simulink model "building_EXAMPLE_v1"  (R2016b)
settings: Solver=ode23tb  StartTime=-building.preruntime+8760*3600  StopTime=building.runtime+8760*3600  MaxStep=600  EnableMultiTasking=on
StartFcn:
  | tic
StopFcn:
  | toc
values from neighbouring files (symbols this model uses):
  building = create_building_automatic(building, modify, import_mode, name_XML, name_EXCEL, name_PHPP, NUMBEROFZONES)    [work_EXAMPLE_v1.m]
undefined symbols (not defined in the file or in its folder): A, B, C, cp, Dd, Dreifach, FluidMix, get_building, ID, MassFlow, p, Pressure, Qdot_C, Qdot_C_energy, Qdot_H, Qdot_H_energy, Qdot_I_electricity, Qdot_I_electricity_energy, Qdot_I_light, Qdot_I_light_energy, Qdot_I_person, Qdot_I_person_energy, Qdot_S, Qdot_S_energy, Qdot_T_ground, Qdot_T_ground_energy, Qdot_T_neighbour, Qdot_T_neighbour_energy, Qdot_T_opaque, Qdot_T_opaque_energy, Qdot_T_window, Qdot_T_window_energy, Qdot_V_infiltration, Qdot_V_infiltration_energy, Qdot_V_mech, Qdot_V_mech_energy, Qdot_V_window, Qdot_V_window_energy, rho, Tc, Temperature, Tr, Ts, Wärmeschutzglas, x_CO2, x_H2O, x_VOC
libraries: carnotUIBK x1931, carnot x83, simulink_extras x22, simulink x12
(part 2 of 35)

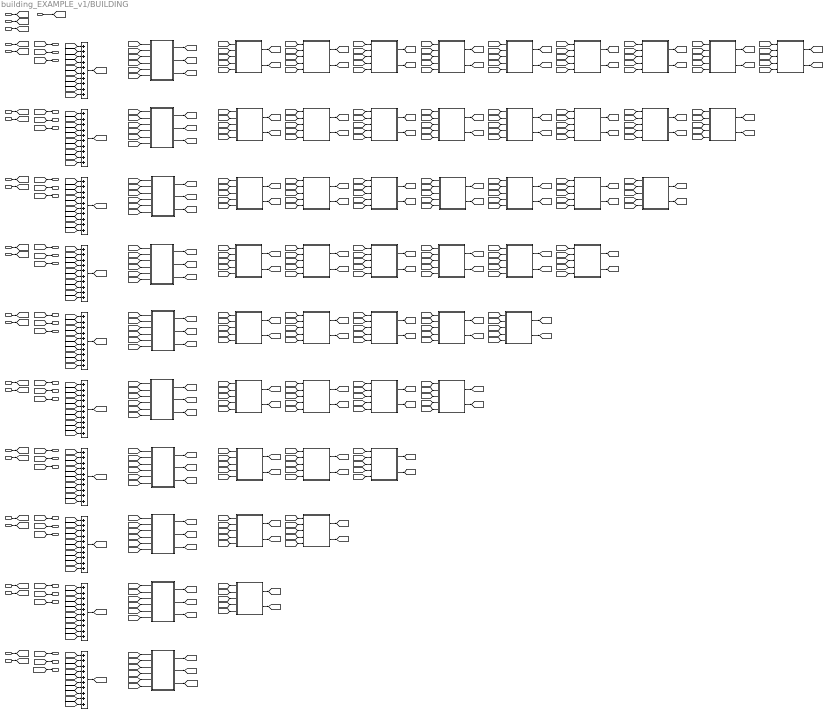
== system building_EXAMPLE_v1/BUILDING ==
  note: INTERSECTION 1_2
  note: ZONE 1 - SUM UP S
  note: ZONE 6 - INPUT AND OUTPUT
  note: ZONE 5 - INPUT AND OUTPUT
  note: ZONE 4 - INPUT AND OUTPUT
  note: ZONE 3 - INPUT AND OUTPUT
  note: ZONE 2 - INPUT AND OUTPUT
  note: ZONE 1 - INPUT AND OUTPUT
  note: BUS BOUNDARY
  note: ZONE 2 - SUM UP S
  note: ZONE 3 - SUM UP S
  note: ZONE 4 - SUM UP S
  note: ZONE 5 - SUM UP S
  note: ZONE 6 - SUM UP S
  note: ZONE 7 - INPUT AND OUTPUT
  note: ZONE 7 - SUM UP S
  note: ZONE 8 - INPUT AND OUTPUT
  note: ZONE 8 - SUM UP S
  note: ZONE 9 - INPUT AND OUTPUT
  note: ZONE 9 - SUM UP S
  note: ZONE 10 - INPUT AND OUTPUT
  note: ZONE 10 - SUM UP S
  note: ZONE 2
  note: ZONE 3
  note: ZONE 4
  note: ZONE 5
  note: ZONE6
  note: ZONE 7
  note: ZONE 8
  note: ZONE 9
  note: ZONE 10
  note: CONTROL
  note: INTERSECTION 1_10
  note: INTERSECTION 1_3
  note: INTERSECTION 1_4
  note: INTERSECTION 1_5
  note: INTERSECTION 1_6
  note: INTERSECTION 1_7
  note: INTERSECTION 1_8
  note: INTERSECTION 1_9
  note: INTERSECTION 2_3
  note: INTERSECTION 2_9
  note: INTERSECTION 2_10
  note: INTERSECTION 2_4
  note: INTERSECTION 2_5
  note: INTERSECTION 2_6
  note: INTERSECTION 2_7
  note: INTERSECTION 2_8
  note: INTERSECTION 3_4
  note: INTERSECTION 3_5
  note: INTERSECTION 3_6
  note: INTERSECTION 3_7
  note: INTERSECTION 3_8
  note: INTERSECTION 3_9
  note: INTERSECTION 3_10
  note: INTERSECTION 4_5
  note: INTERSECTION 4_6
  note: INTERSECTION 4_7
  note: INTERSECTION 4_8
  note: INTERSECTION 4_9
  note: INTERSECTION 4_10
  note: INTERSECTION 5_6
  note: INTERSECTION 5_7
  note: INTERSECTION 5_8
  note: INTERSECTION 5_9
  note: INTERSECTION 5_10
  note: INTERSECTION 6_7
  note: INTERSECTION 6_8
  note: INTERSECTION 6_9
  note: INTERSECTION 6_10
  note: INTERSECTION 7_8
  note: INTERSECTION 7_9
  note: INTERSECTION 7_10
  note: INTERSECTION 8_9
  note: INTERSECTION 8_10
  note: INTERSECTION 9_10
  note: ZONE 1
  WDB : Inport
  GDB : Inport  Port=2
  NDB : Inport  Port=3
  S_HVAC[1] : Inport  Port=4
  qdot_in[1] : Inport  Port=5
  S_HVAC[2] : Inport  Port=6
  qdot_in[2] : Inport  Port=7
  S_HVAC[3] : Inport  Port=8
  qdot_in[3] : Inport  Port=9
  S_HVAC[4] : Inport  Port=10
  qdot_in[4] : Inport  Port=11
  S_HVAC[5] : Inport  Port=12
  qdot_in[5] : Inport  Port=13
  S_HVAC[6] : Inport  Port=14
  qdot_in[6] : Inport  Port=15
  S_HVAC[7] : Inport  Port=16
  qdot_in[7] : Inport  Port=17
  S_HVAC[8] : Inport  Port=18
  qdot_in[8] : Inport  Port=19
  S_HVAC[9] : Inport  Port=20
  qdot_in[9] : Inport  Port=21
  S_HVAC[10] : Inport  Port=22
  qdot_in[10] : Inport  Port=23
  control : Inport  Port=24
  Add{,1..9} (10 alike) : Sum  Inputs=++++++++++
  INTERSECTION_1_10 : Subsystem  VariantControl=Variant1  mask{intersection=b.thermalzone.intersection{1,10}}
      mask prompts: intersection "INTERSECTION object"
      mask init:
      | i = intersection;
      | z = intersection;
      mask Display: fprintf('%s',intersection.name)
  INTERSECTION_1_2 : Subsystem  VariantControl=Variant1  mask{intersection=b.thermalzone.intersection{1,2}}
      mask prompts: intersection "INTERSECTION object"
      mask init:
      | i = intersection;
      | z = intersection;
      mask Display: fprintf('%s',intersection.name)
  INTERSECTION_1_3 : Subsystem  VariantControl=Variant1  mask{intersection=b.thermalzone.intersection{1,3}}
      mask prompts: intersection "INTERSECTION object"
      mask init:
      | i = intersection;
      | z = intersection;
      mask Display: fprintf('%s',intersection.name)
  INTERSECTION_1_4 : Subsystem  VariantControl=Variant1  mask{intersection=b.thermalzone.intersection{1,4}}
      mask prompts: intersection "INTERSECTION object"
      mask init:
      | i = intersection;
      | z = intersection;
      mask Display: fprintf('%s',intersection.name)
  INTERSECTION_1_5 : Subsystem  VariantControl=Variant1  mask{intersection=b.thermalzone.intersection{1,5}}
      mask prompts: intersection "INTERSECTION object"
      mask init:
      | i = intersection;
      | z = intersection;
      mask Display: fprintf('%s',intersection.name)
  INTERSECTION_1_6 : Subsystem  VariantControl=Variant1  mask{intersection=b.thermalzone.intersection{1,6}}
      mask prompts: intersection "INTERSECTION object"
      mask init:
      | i = intersection;
      | z = intersection;
      mask Display: fprintf('%s',intersection.name)
  INTERSECTION_1_7 : Subsystem  VariantControl=Variant1  mask{intersection=b.thermalzone.intersection{1,7}}
      mask prompts: intersection "INTERSECTION object"
      mask init:
      | i = intersection;
      | z = intersection;
      mask Display: fprintf('%s',intersection.name)
  INTERSECTION_1_8 : Subsystem  VariantControl=Variant1  mask{intersection=b.thermalzone.intersection{1,8}}
      mask prompts: intersection "INTERSECTION object"
      mask init:
      | i = intersection;
      | z = intersection;
      mask Display: fprintf('%s',intersection.name)
  INTERSECTION_1_9 : Subsystem  VariantControl=Variant1  mask{intersection=b.thermalzone.intersection{1,9}}
      mask prompts: intersection "INTERSECTION object"
      mask init:
      | i = intersection;
      | z = intersection;
      mask Display: fprintf('%s',intersection.name)
  INTERSECTION_2_10 : Subsystem  VariantControl=Variant1  mask{intersection=b.thermalzone.intersection{2,10}}
      mask prompts: intersection "INTERSECTION object"
      mask init:
      | i = intersection;
      | z = intersection;
      mask Display: fprintf('%s',intersection.name)
  INTERSECTION_2_3 : Subsystem  VariantControl=Variant1  mask{intersection=b.thermalzone.intersection{2,3}}
      mask prompts: intersection "INTERSECTION object"
      mask init:
      | i = intersection;
      | z = intersection;
      mask Display: fprintf('%s',intersection.name)
  INTERSECTION_2_4 : Subsystem  VariantControl=Variant1  mask{intersection=b.thermalzone.intersection{2,4}}
      mask prompts: intersection "INTERSECTION object"
      mask init:
      | i = intersection;
      | z = intersection;
      mask Display: fprintf('%s',intersection.name)
  INTERSECTION_2_5 : Subsystem  VariantControl=Variant1  mask{intersection=b.thermalzone.intersection{2,5}}
      mask prompts: intersection "INTERSECTION object"
      mask init:
      | i = intersection;
      | z = intersection;
      mask Display: fprintf('%s',intersection.name)
  INTERSECTION_2_6 : Subsystem  VariantControl=Variant1  mask{intersection=b.thermalzone.intersection{2,6}}
      mask prompts: intersection "INTERSECTION object"
      mask init:
      | i = intersection;
      | z = intersection;
      mask Display: fprintf('%s',intersection.name)
  INTERSECTION_2_7 : Subsystem  VariantControl=Variant1  mask{intersection=b.thermalzone.intersection{2,7}}
      mask prompts: intersection "INTERSECTION object"
      mask init:
      | i = intersection;
      | z = intersection;
      mask Display: fprintf('%s',intersection.name)
  INTERSECTION_2_8 : Subsystem  VariantControl=Variant1  mask{intersection=b.thermalzone.intersection{2,8}}
      mask prompts: intersection "INTERSECTION object"
      mask init:
      | i = intersection;
      | z = intersection;
      mask Display: fprintf('%s',intersection.name)
  INTERSECTION_2_9 : Subsystem  VariantControl=Variant1  mask{intersection=b.thermalzone.intersection{2,9}}
      mask prompts: intersection "INTERSECTION object"
      mask init:
      | i = intersection;
      | z = intersection;
      mask Display: fprintf('%s',intersection.name)
  INTERSECTION_3_10 : Subsystem  VariantControl=Variant1  mask{intersection=b.thermalzone.intersection{3,10}}
      mask prompts: intersection "INTERSECTION object"
      mask init:
      | i = intersection;
      | z = intersection;
      mask Display: fprintf('%s',intersection.name)
  INTERSECTION_3_4 : Subsystem  VariantControl=Variant1  mask{intersection=b.thermalzone.intersection{3,4}}
      mask prompts: intersection "INTERSECTION object"
      mask init:
      | i = intersection;
      | z = intersection;
      mask Display: fprintf('%s',intersection.name)
  INTERSECTION_3_5 : Subsystem  VariantControl=Variant1  mask{intersection=b.thermalzone.intersection{3,5}}
      mask prompts: intersection "INTERSECTION object"
      mask init:
      | i = intersection;
      | z = intersection;
      mask Display: fprintf('%s',intersection.name)
  INTERSECTION_3_6 : Subsystem  VariantControl=Variant1  mask{intersection=b.thermalzone.intersection{3,6}}
      mask prompts: intersection "INTERSECTION object"
      mask init:
      | i = intersection;
      | z = intersection;
      mask Display: fprintf('%s',intersection.name)
  INTERSECTION_3_7 : Subsystem  VariantControl=Variant1  mask{intersection=b.thermalzone.intersection{3,7}}
      mask prompts: intersection "INTERSECTION object"
      mask init:
      | i = intersection;
      | z = intersection;
      mask Display: fprintf('%s',intersection.name)
  INTERSECTION_3_8 : Subsystem  VariantControl=Variant1  mask{intersection=b.thermalzone.intersection{3,8}}
      mask prompts: intersection "INTERSECTION object"
      mask init:
      | i = intersection;
      | z = intersection;
      mask Display: fprintf('%s',intersection.name)
  INTERSECTION_3_9 : Subsystem  VariantControl=Variant1  mask{intersection=b.thermalzone.intersection{3,9}}
      mask prompts: intersection "INTERSECTION object"
      mask init:
      | i = intersection;
      | z = intersection;
      mask Display: fprintf('%s',intersection.name)
  INTERSECTION_4_10 : Subsystem  VariantControl=Variant1  mask{intersection=b.thermalzone.intersection{4,10}}
      mask prompts: intersection "INTERSECTION object"
      mask init:
      | i = intersection;
      | z = intersection;
      mask Display: fprintf('%s',intersection.name)
  INTERSECTION_4_5 : Subsystem  VariantControl=Variant1  mask{intersection=b.thermalzone.intersection{4,5}}
      mask prompts: intersection "INTERSECTION object"
      mask init:
      | i = intersection;
      | z = intersection;
      mask Display: fprintf('%s',intersection.name)
  INTERSECTION_4_6 : Subsystem  VariantControl=Variant1  mask{intersection=b.thermalzone.intersection{4,6}}
      mask prompts: intersection "INTERSECTION object"
      mask init:
      | i = intersection;
      | z = intersection;
      mask Display: fprintf('%s',intersection.name)
  INTERSECTION_4_7 : Subsystem  VariantControl=Variant1  mask{intersection=b.thermalzone.intersection{4,7}}
      mask prompts: intersection "INTERSECTION object"
      mask init:
      | i = intersection;
      | z = intersection;
      mask Display: fprintf('%s',intersection.name)
  INTERSECTION_4_8 : Subsystem  VariantControl=Variant1  mask{intersection=b.thermalzone.intersection{4,8}}
      mask prompts: intersection "INTERSECTION object"
      mask init:
      | i = intersection;
      | z = intersection;
      mask Display: fprintf('%s',intersection.name)
  INTERSECTION_4_9 : Subsystem  VariantControl=Variant1  mask{intersection=b.thermalzone.intersection{4,9}}
      mask prompts: intersection "INTERSECTION object"
      mask init:
      | i = intersection;
      | z = intersection;
      mask Display: fprintf('%s',intersection.name)
  INTERSECTION_5_10 : Subsystem  VariantControl=Variant1  mask{intersection=b.thermalzone.intersection{5,10}}
      mask prompts: intersection "INTERSECTION object"
      mask init:
      | i = intersection;
      | z = intersection;
      mask Display: fprintf('%s',intersection.name)
  INTERSECTION_5_6 : Subsystem  VariantControl=Variant1  mask{intersection=b.thermalzone.intersection{5,6}}
      mask prompts: intersection "INTERSECTION object"
      mask init:
      | i = intersection;
      | z = intersection;
      mask Display: fprintf('%s',intersection.name)
  INTERSECTION_5_7 : Subsystem  VariantControl=Variant1  mask{intersection=b.thermalzone.intersection{5,7}}
      mask prompts: intersection "INTERSECTION object"
      mask init:
      | i = intersection;
      | z = intersection;
      mask Display: fprintf('%s',intersection.name)
  INTERSECTION_5_8 : Subsystem  VariantControl=Variant1  mask{intersection=b.thermalzone.intersection{5,8}}
      mask prompts: intersection "INTERSECTION object"
      mask init:
      | i = intersection;
      | z = intersection;
      mask Display: fprintf('%s',intersection.name)
  INTERSECTION_5_9 : Subsystem  VariantControl=Variant1  mask{intersection=b.thermalzone.intersection{5,9}}
      mask prompts: intersection "INTERSECTION object"
      mask init:
      | i = intersection;
      | z = intersection;
      mask Display: fprintf('%s',intersection.name)
  INTERSECTION_6_10 : Subsystem  VariantControl=Variant1  mask{intersection=b.thermalzone.intersection{6,10}}
      mask prompts: intersection "INTERSECTION object"
      mask init:
      | i = intersection;
      | z = intersection;
      mask Display: fprintf('%s',intersection.name)
  INTERSECTION_6_7 : Subsystem  VariantControl=Variant1  mask{intersection=b.thermalzone.intersection{6,7}}
      mask prompts: intersection "INTERSECTION object"
      mask init:
      | i = intersection;
      | z = intersection;
      mask Display: fprintf('%s',intersection.name)
  INTERSECTION_6_8 : Subsystem  VariantControl=Variant1  mask{intersection=b.thermalzone.intersection{6,8}}
      mask prompts: intersection "INTERSECTION object"
      mask init:
      | i = intersection;
      | z = intersection;
      mask Display: fprintf('%s',intersection.name)
  INTERSECTION_6_9 : Subsystem  VariantControl=Variant1  mask{intersection=b.thermalzone.intersection{6,9}}
      mask prompts: intersection "INTERSECTION object"
      mask init:
      | i = intersection;
      | z = intersection;
      mask Display: fprintf('%s',intersection.name)
  INTERSECTION_7_10 : Subsystem  VariantControl=Variant1  mask{intersection=b.thermalzone.intersection{7,10}}
      mask prompts: intersection "INTERSECTION object"
      mask init:
      | i = intersection;
      | z = intersection;
      mask Display: fprintf('%s',intersection.name)
  INTERSECTION_7_8 : Subsystem  VariantControl=Variant1  mask{intersection=b.thermalzone.intersection{7,8}}
      mask prompts: intersection "INTERSECTION object"
      mask init:
      | i = intersection;
      | z = intersection;
      mask Display: fprintf('%s',intersection.name)
  INTERSECTION_7_9 : Subsystem  VariantControl=Variant1  mask{intersection=b.thermalzone.intersection{7,9}}
      mask prompts: intersection "INTERSECTION object"
      mask init:
      | i = intersection;
      | z = intersection;
      mask Display: fprintf('%s',intersection.name)
  INTERSECTION_8_10 : Subsystem  VariantControl=Variant1  mask{intersection=b.thermalzone.intersection{8,10}}
      mask prompts: intersection "INTERSECTION object"
      mask init:
      | i = intersection;
      | z = intersection;
      mask Display: fprintf('%s',intersection.name)
  INTERSECTION_8_9 : Subsystem  VariantControl=Variant1  mask{intersection=b.thermalzone.intersection{8,9}}
      mask prompts: intersection "INTERSECTION object"
      mask init:
      | i = intersection;
      | z = intersection;
      mask Display: fprintf('%s',intersection.name)
  INTERSECTION_9_10 : Subsystem  VariantControl=Variant1  mask{intersection=b.thermalzone.intersection{9,10}}
      mask prompts: intersection "INTERSECTION object"
      mask init:
      | i = intersection;
      | z = intersection;
      mask Display: fprintf('%s',intersection.name)
  ZONE_1 : Subsystem  mask{zone=b.thermalzone.zone(1)}
      mask prompts: zone "ZONE object"
      mask init:
      | z = zone;
      mask Display: fprintf('%s',zone.name)
  ZONE_10 : Subsystem  mask{zone=b.thermalzone.zone(10)}
      mask prompts: zone "ZONE object"
      mask init:
      | z = zone;
      mask Display: fprintf('%s',zone.name)
  ZONE_2 : Subsystem  mask{zone=b.thermalzone.zone(2)}
      mask prompts: zone "ZONE object"
      mask init:
      | z = zone;
      mask Display: fprintf('%s',zone.name)
  ZONE_3 : Subsystem  mask{zone=b.thermalzone.zone(3)}
      mask prompts: zone "ZONE object"
      mask init:
      | z = zone;
      mask Display: fprintf('%s',zone.name)
  ZONE_4 : Subsystem  mask{zone=b.thermalzone.zone(4)}
      mask prompts: zone "ZONE object"
      mask init:
      | z = zone;
      mask Display: fprintf('%s',zone.name)
  ZONE_5 : Subsystem  mask{zone=b.thermalzone.zone(5)}
      mask prompts: zone "ZONE object"
      mask init:
      | z = zone;
      mask Display: fprintf('%s',zone.name)
  ZONE_6 : Subsystem  mask{zone=b.thermalzone.zone(6)}
      mask prompts: zone "ZONE object"
      mask init:
      | z = zone;
      mask Display: fprintf('%s',zone.name)
  ZONE_7 : Subsystem  mask{zone=b.thermalzone.zone(7)}
      mask prompts: zone "ZONE object"
      mask init:
      | z = zone;
      mask Display: fprintf('%s',zone.name)
  ZONE_8 : Subsystem  mask{zone=b.thermalzone.zone(8)}
      mask prompts: zone "ZONE object"
      mask init:
      | z = zone;
      mask Display: fprintf('%s',zone.name)
  ZONE_9 : Subsystem  mask{zone=b.thermalzone.zone(9)}
      mask prompts: zone "ZONE object"
      mask init:
      | z = zone;
      mask Display: fprintf('%s',zone.name)
  BDB[1] : Outport
  AIB[1] : Outport  Port=2
  theta_out[1] : Outport  Port=3
  BDB[2] : Outport  Port=4
  AIB[2] : Outport  Port=5
  theta_out[2] : Outport  Port=6
  BDB[3] : Outport  Port=7
  AIB[3] : Outport  Port=8
  theta_out[3] : Outport  Port=9
  BDB[4] : Outport  Port=10
  AIB[4] : Outport  Port=11
  theta_out[4] : Outport  Port=12
  BDB[5] : Outport  Port=13
  AIB[5] : Outport  Port=14
  theta_out[5] : Outport  Port=15
  BDB[6] : Outport  Port=16
  AIB[6] : Outport  Port=17
  theta_out[6] : Outport  Port=18
  BDB[7] : Outport  Port=19
  AIB[7] : Outport  Port=20
  theta_out[7] : Outport  Port=21
  BDB[8] : Outport  Port=22
  AIB[8] : Outport  Port=23
  theta_out[8] : Outport  Port=24
  BDB[9] : Outport  Port=25
  AIB[9] : Outport  Port=26
  theta_out[9] : Outport  Port=27
  BDB[10] : Outport  Port=28
  AIB[10] : Outport  Port=29
  theta_out[10] : Outport  Port=30
  wires:
  WDB/1 -> [WDB]
  GDB/1 -> [GDB]
  NDB/1 -> [NDB]
  S_HVAC[1]/1 -> [S_HVAC_1]
  qdot_in[1]/1 -> [qdot_in_1]
  [BDB_1] -> BDB[1]/1
  [AIB_1] -> AIB[1]/1
  [theta_out_1] -> theta_out[1]/1
  S_HVAC[2]/1 -> [S_HVAC_2]
  qdot_in[2]/1 -> [qdot_in_2]
  qdot_in[3]/1 -> [qdot_in_3]
  S_HVAC[3]/1 -> [S_HVAC_3]
  S_HVAC[4]/1 -> [S_HVAC_4]
  qdot_in[4]/1 -> [qdot_in_4]
  S_HVAC[5]/1 -> [S_HVAC_5]
  qdot_in[5]/1 -> [qdot_in_5]
  qdot_in[6]/1 -> [qdot_in_6]
  S_HVAC[6]/1 -> [S_HVAC_6]
  [BDB_2] -> BDB[2]/1
  [AIB_2] -> AIB[2]/1
  [theta_out_2] -> theta_out[2]/1
  [BDB_3] -> BDB[3]/1
  [AIB_3] -> AIB[3]/1
  [theta_out_3] -> theta_out[3]/1
  [BDB_4] -> BDB[4]/1
  [AIB_4] -> AIB[4]/1
  [theta_out_4] -> theta_out[4]/1
  [BDB_5] -> BDB[5]/1
  [AIB_5] -> AIB[5]/1
  [theta_out_5] -> theta_out[5]/1
  [BDB_6] -> BDB[6]/1
  [AIB_6] -> AIB[6]/1
  [theta_out_6] -> theta_out[6]/1
  [S_HVAC_1] -> Add/1
  [S_I_16] -> Add/6
  [S_I_12] -> Add/2
  [S_I_13] -> Add/3
  [S_I_14] -> Add/4
  [S_I_15] -> Add/5
  Add/1 -> [S_in_1]
  [S_HVAC_2] -> Add1/1
  Add1/1 -> [S_in_2]
  Add2/1 -> [S_in_3]
  Add3/1 -> [S_in_4]
  Add4/1 -> [S_in_5]
  Add5/1 -> [S_in_6]
  [S_I_17] -> Add/7
  [S_I_18] -> Add/8
  [S_I_19] -> Add/9
  [S_I_110] -> Add/10
  [S_I_27] -> Add1/7
  [S_I_28] -> Add1/8
  [S_I_29] -> Add1/9
  [S_I_210] -> Add1/10
  [S_I_21] -> Add1/2
  [S_I_23] -> Add1/3
  [S_I_26] -> Add1/6
  [S_I_25] -> Add1/5
  [S_I_24] -> Add1/4
  [S_I_37] -> Add2/7
  [S_I_38] -> Add2/8
  [S_I_39] -> Add2/9
  [S_I_310] -> Add2/10
  [S_HVAC_3] -> Add2/1
  [S_I_31] -> Add2/2
  [S_I_32] -> Add2/3
  [S_I_34] -> Add2/4
  [S_I_35] -> Add2/5
  [S_I_36] -> Add2/6
  [S_I_47] -> Add3/7
  [S_I_48] -> Add3/8
  [S_I_49] -> Add3/9
  [S_I_410] -> Add3/10
  [S_HVAC_4] -> Add3/1
  [S_I_41] -> Add3/2
  [S_I_42] -> Add3/3
  [S_I_43] -> Add3/4
  [S_I_45] -> Add3/5
  [S_I_46] -> Add3/6
  [S_I_57] -> Add4/7
  [S_I_58] -> Add4/8
  [S_I_59] -> Add4/9
  [S_I_510] -> Add4/10
  [S_HVAC_5] -> Add4/1
  [S_I_51] -> Add4/2
  [S_I_52] -> Add4/3
  [S_I_53] -> Add4/4
  [S_I_54] -> Add4/5
  [S_I_56] -> Add4/6
  [S_I_67] -> Add5/7
  [S_I_68] -> Add5/8
  [S_I_69] -> Add5/9
  [S_I_610] -> Add5/10
  [S_HVAC_6] -> Add5/1
  [S_I_61] -> Add5/2
  [S_I_62] -> Add5/3
  [S_I_63] -> Add5/4
  [S_I_64] -> Add5/5
  [S_I_65] -> Add5/6
  qdot_in[7]/1 -> [qdot_in_7]
  S_HVAC[7]/1 -> [S_HVAC_7]
  [BDB_7] -> BDB[7]/1
  [AIB_7] -> AIB[7]/1
  [theta_out_7] -> theta_out[7]/1
  Add6/1 -> [S_in_7]
  [S_I_76] -> Add6/7
  [S_I_78] -> Add6/8
  [S_I_79] -> Add6/9
  [S_I_710] -> Add6/10
  [S_HVAC_7] -> Add6/1
  [S_I_71] -> Add6/2
  [S_I_72] -> Add6/3
  [S_I_73] -> Add6/4
  [S_I_74] -> Add6/5
  [S_I_75] -> Add6/6
  qdot_in[8]/1 -> [qdot_in_8]
  S_HVAC[8]/1 -> [S_HVAC_8]
  [BDB_8] -> BDB[8]/1
  [AIB_8] -> AIB[8]/1
  [theta_out_8] -> theta_out[8]/1
  Add7/1 -> [S_in_8]
  [S_I_86] -> Add7/7
  [S_I_87] -> Add7/8
  [S_I_89] -> Add7/9
  [S_I_810] -> Add7/10
  [S_HVAC_8] -> Add7/1
  [S_I_81] -> Add7/2
  [S_I_82] -> Add7/3
  [S_I_83] -> Add7/4
  [S_I_84] -> Add7/5
  [S_I_85] -> Add7/6
  qdot_in[9]/1 -> [qdot_in_9]
  S_HVAC[9]/1 -> [S_HVAC_9]
  [BDB_9] -> BDB[9]/1
  [AIB_9] -> AIB[9]/1
  [theta_out_9] -> theta_out[9]/1
  Add8/1 -> [S_in_9]
  [S_I_96] -> Add8/7
  [S_I_97] -> Add8/8
  [S_I_98] -> Add8/9
  [S_I_910] -> Add8/10
  [S_HVAC_9] -> Add8/1
  [S_I_91] -> Add8/2
  [S_I_92] -> Add8/3
  [S_I_93] -> Add8/4
  [S_I_94] -> Add8/5
  [S_I_95] -> Add8/6
  qdot_in[10]/1 -> [qdot_in_10]
  S_HVAC[10]/1 -> [S_HVAC_10]
  [BDB_10] -> BDB[10]/1
  [AIB_10] -> AIB[10]/1
  [theta_out_10] -> theta_out[10]/1
  Add9/1 -> [S_in_10]
  [S_I_106] -> Add9/7
  [S_I_107] -> Add9/8
  [S_I_108] -> Add9/9
  [S_I_109] -> Add9/10
  [S_HVAC_10] -> Add9/1
  [S_I_101] -> Add9/2
  [S_I_102] -> Add9/3
  [S_I_103] -> Add9/4
  [S_I_104] -> Add9/5
  [S_I_105] -> Add9/6
  ZONE_2/1(BDB) -> [BDB_2]
  ZONE_2/2(AIB) -> [AIB_2]
  ZONE_2/3(theta_out) -> [theta_out_2z]
  [qdot_in_2] -> ZONE_2/5(Qdot_in)
  [S_in_2] -> ZONE_2/4(S_in)
  [GDB] -> ZONE_2/2(GDB)
  [WDB] -> ZONE_2/1(WDB)
  [NDB] -> ZONE_2/3(NDB)
  ZONE_3/1(BDB) -> [BDB_3]
  ZONE_3/2(AIB) -> [AIB_3]
  ZONE_3/3(theta_out) -> [theta_out_3z]
  [qdot_in_3] -> ZONE_3/5(Qdot_in)
  [S_in_3] -> ZONE_3/4(S_in)
  [GDB] -> ZONE_3/2(GDB)
  [WDB] -> ZONE_3/1(WDB)
  [NDB] -> ZONE_3/3(NDB)
  ZONE_4/1(BDB) -> [BDB_4]
  ZONE_4/2(AIB) -> [AIB_4]
  ZONE_4/3(theta_out) -> [theta_out_4z]
  [qdot_in_4] -> ZONE_4/5(Qdot_in)
  [S_in_4] -> ZONE_4/4(S_in)
  [GDB] -> ZONE_4/2(GDB)
  [WDB] -> ZONE_4/1(WDB)
  [NDB] -> ZONE_4/3(NDB)
  ZONE_5/1(BDB) -> [BDB_5]
  ZONE_5/2(AIB) -> [AIB_5]
  ZONE_5/3(theta_out) -> [theta_out_5z]
  [qdot_in_5] -> ZONE_5/5(Qdot_in)
  [S_in_5] -> ZONE_5/4(S_in)
  [GDB] -> ZONE_5/2(GDB)
  [WDB] -> ZONE_5/1(WDB)
  [NDB] -> ZONE_5/3(NDB)
  ZONE_6/1(BDB) -> [BDB_6]
  ZONE_6/2(AIB) -> [AIB_6]
  ZONE_6/3(theta_out) -> [theta_out_6z]
  [qdot_in_6] -> ZONE_6/5(Qdot_in)
  [S_in_6] -> ZONE_6/4(S_in)
  [GDB] -> ZONE_6/2(GDB)
  [WDB] -> ZONE_6/1(WDB)
  [NDB] -> ZONE_6/3(NDB)
  ZONE_7/1(BDB) -> [BDB_7]
  ZONE_7/2(AIB) -> [AIB_7]
  ZONE_7/3(theta_out) -> [theta_out_7z]
  [qdot_in_7] -> ZONE_7/5(Qdot_in)
  [S_in_7] -> ZONE_7/4(S_in)
  [GDB] -> ZONE_7/2(GDB)
  [WDB] -> ZONE_7/1(WDB)
  [NDB] -> ZONE_7/3(NDB)
  ZONE_8/1(BDB) -> [BDB_8]
  ZONE_8/2(AIB) -> [AIB_8]
  ZONE_8/3(theta_out) -> [theta_out_8z]
  [qdot_in_8] -> ZONE_8/5(Qdot_in)
  [S_in_8] -> ZONE_8/4(S_in)
  [GDB] -> ZONE_8/2(GDB)
  [WDB] -> ZONE_8/1(WDB)
  [NDB] -> ZONE_8/3(NDB)
  ZONE_9/1(BDB) -> [BDB_9]
  ZONE_9/2(AIB) -> [AIB_9]
  ZONE_9/3(theta_out) -> [theta_out_9z]
  [qdot_in_9] -> ZONE_9/5(Qdot_in)
  [S_in_9] -> ZONE_9/4(S_in)
  [GDB] -> ZONE_9/2(GDB)
  [WDB] -> ZONE_9/1(WDB)
  [NDB] -> ZONE_9/3(NDB)
  ZONE_10/1(BDB) -> [BDB_10]
  ZONE_10/2(AIB) -> [AIB_10]
  ZONE_10/3(theta_out) -> [theta_out_10z]
  [qdot_in_10] -> ZONE_10/5(Qdot_in)
  [S_in_10] -> ZONE_10/4(S_in)
  [GDB] -> ZONE_10/2(GDB)
  [WDB] -> ZONE_10/1(WDB)
  [NDB] -> ZONE_10/3(NDB)
  control/1 -> [control]
  [AIB_1] -> INTERSECTION_1_2/1(AIB1)
  [AIB_2] -> INTERSECTION_1_2/2(AIB2)
  INTERSECTION_1_2/1(S1) -> [S_I_12]
  INTERSECTION_1_2/2(S2) -> [S_I_21]
  [control] -> ZONE_2/6(control)
  [control] -> ZONE_3/6(control)
  [control] -> ZONE_4/6(control)
  [control] -> ZONE_5/6(control)
  [control] -> ZONE_6/6(control)
  [control] -> ZONE_7/6(control)
  [control] -> ZONE_8/6(control)
  [control] -> ZONE_9/6(control)
  [control] -> ZONE_10/6(control)
  [BDB_1] -> INTERSECTION_1_2/3(BDB1)
  [BDB_2] -> INTERSECTION_1_2/4(BDB2)
  [control] -> INTERSECTION_1_2/5(control)
  [AIB_1] -> INTERSECTION_1_10/1(AIB1)
  [AIB_10] -> INTERSECTION_1_10/2(AIB2)
  INTERSECTION_1_10/1(S1) -> [S_I_110]
  INTERSECTION_1_10/2(S2) -> [S_I_101]
  [BDB_1] -> INTERSECTION_1_10/3(BDB1)
  [BDB_10] -> INTERSECTION_1_10/4(BDB2)
  [control] -> INTERSECTION_1_10/5(control)
  [AIB_1] -> INTERSECTION_1_3/1(AIB1)
  [AIB_3] -> INTERSECTION_1_3/2(AIB2)
  INTERSECTION_1_3/1(S1) -> [S_I_13]
  INTERSECTION_1_3/2(S2) -> [S_I_31]
  [BDB_1] -> INTERSECTION_1_3/3(BDB1)
  [BDB_3] -> INTERSECTION_1_3/4(BDB2)
  [control] -> INTERSECTION_1_3/5(control)
  [AIB_1] -> INTERSECTION_1_4/1(AIB1)
  [AIB_4] -> INTERSECTION_1_4/2(AIB2)
  INTERSECTION_1_4/1(S1) -> [S_I_14]
  INTERSECTION_1_4/2(S2) -> [S_I_41]
  [BDB_1] -> INTERSECTION_1_4/3(BDB1)
  [BDB_4] -> INTERSECTION_1_4/4(BDB2)
  [control] -> INTERSECTION_1_4/5(control)
  [AIB_1] -> INTERSECTION_1_5/1(AIB1)
  [AIB_5] -> INTERSECTION_1_5/2(AIB2)
  INTERSECTION_1_5/1(S1) -> [S_I_15]
  INTERSECTION_1_5/2(S2) -> [S_I_51]
  [BDB_1] -> INTERSECTION_1_5/3(BDB1)
  [BDB_5] -> INTERSECTION_1_5/4(BDB2)
  [control] -> INTERSECTION_1_5/5(control)
  [AIB_1] -> INTERSECTION_1_6/1(AIB1)
  [AIB_6] -> INTERSECTION_1_6/2(AIB2)
  INTERSECTION_1_6/1(S1) -> [S_I_16]
  INTERSECTION_1_6/2(S2) -> [S_I_61]
  [BDB_1] -> INTERSECTION_1_6/3(BDB1)
  [BDB_6] -> INTERSECTION_1_6/4(BDB2)
  [control] -> INTERSECTION_1_6/5(control)
  [AIB_1] -> INTERSECTION_1_7/1(AIB1)
  [AIB_7] -> INTERSECTION_1_7/2(AIB2)
  INTERSECTION_1_7/1(S1) -> [S_I_17]
  INTERSECTION_1_7/2(S2) -> [S_I_71]
  [BDB_1] -> INTERSECTION_1_7/3(BDB1)
  [BDB_7] -> INTERSECTION_1_7/4(BDB2)
  [control] -> INTERSECTION_1_7/5(control)
  [AIB_1] -> INTERSECTION_1_8/1(AIB1)
  [AIB_8] -> INTERSECTION_1_8/2(AIB2)
  INTERSECTION_1_8/1(S1) -> [S_I_18]
  INTERSECTION_1_8/2(S2) -> [S_I_81]
  [BDB_1] -> INTERSECTION_1_8/3(BDB1)
  [BDB_8] -> INTERSECTION_1_8/4(BDB2)
  [control] -> INTERSECTION_1_8/5(control)
  [AIB_1] -> INTERSECTION_1_9/1(AIB1)
  [AIB_9] -> INTERSECTION_1_9/2(AIB2)
  INTERSECTION_1_9/1(S1) -> [S_I_19]
  INTERSECTION_1_9/2(S2) -> [S_I_91]
  [BDB_1] -> INTERSECTION_1_9/3(BDB1)
  [BDB_9] -> INTERSECTION_1_9/4(BDB2)
  [control] -> INTERSECTION_1_9/5(control)
  [AIB_2] -> INTERSECTION_2_3/1(AIB1)
  [AIB_3] -> INTERSECTION_2_3/2(AIB2)
  INTERSECTION_2_3/1(S1) -> [S_I_23]
  INTERSECTION_2_3/2(S2) -> [S_I_32]
  [BDB_2] -> INTERSECTION_2_3/3(BDB1)
  [BDB_3] -> INTERSECTION_2_3/4(BDB2)
  [control] -> INTERSECTION_2_3/5(control)
  [AIB_2] -> INTERSECTION_2_9/1(AIB1)
  [AIB_9] -> INTERSECTION_2_9/2(AIB2)
  INTERSECTION_2_9/1(S1) -> [S_I_29]
  INTERSECTION_2_9/2(S2) -> [S_I_92]
  [BDB_2] -> INTERSECTION_2_9/3(BDB1)
  [BDB_9] -> INTERSECTION_2_9/4(BDB2)
  [control] -> INTERSECTION_2_9/5(control)
  [AIB_2] -> INTERSECTION_2_10/1(AIB1)
  [AIB_10] -> INTERSECTION_2_10/2(AIB2)
  INTERSECTION_2_10/1(S1) -> [S_I_210]
  INTERSECTION_2_10/2(S2) -> [S_I_102]
  [BDB_2] -> INTERSECTION_2_10/3(BDB1)
  [BDB_10] -> INTERSECTION_2_10/4(BDB2)
  [control] -> INTERSECTION_2_10/5(control)
  [AIB_2] -> INTERSECTION_2_4/1(AIB1)
  [AIB_4] -> INTERSECTION_2_4/2(AIB2)
  INTERSECTION_2_4/1(S1) -> [S_I_24]
  INTERSECTION_2_4/2(S2) -> [S_I_42]
  [BDB_2] -> INTERSECTION_2_4/3(BDB1)
  [BDB_4] -> INTERSECTION_2_4/4(BDB2)
  [control] -> INTERSECTION_2_4/5(control)
  [AIB_2] -> INTERSECTION_2_5/1(AIB1)
  [AIB_5] -> INTERSECTION_2_5/2(AIB2)
  INTERSECTION_2_5/1(S1) -> [S_I_25]
  INTERSECTION_2_5/2(S2) -> [S_I_52]
  [BDB_2] -> INTERSECTION_2_5/3(BDB1)
  [BDB_5] -> INTERSECTION_2_5/4(BDB2)
  [control] -> INTERSECTION_2_5/5(control)
  [AIB_2] -> INTERSECTION_2_6/1(AIB1)
  [AIB_6] -> INTERSECTION_2_6/2(AIB2)
  INTERSECTION_2_6/1(S1) -> [S_I_26]
  INTERSECTION_2_6/2(S2) -> [S_I_62]
  [BDB_2] -> INTERSECTION_2_6/3(BDB1)
  [BDB_6] -> INTERSECTION_2_6/4(BDB2)
  [control] -> INTERSECTION_2_6/5(control)
  [AIB_2] -> INTERSECTION_2_7/1(AIB1)
  [AIB_7] -> INTERSECTION_2_7/2(AIB2)
  INTERSECTION_2_7/1(S1) -> [S_I_27]
  INTERSECTION_2_7/2(S2) -> [S_I_72]
  [BDB_2] -> INTERSECTION_2_7/3(BDB1)
  [BDB_7] -> INTERSECTION_2_7/4(BDB2)
  [control] -> INTERSECTION_2_7/5(control)
  [AIB_2] -> INTERSECTION_2_8/1(AIB1)
  [AIB_8] -> INTERSECTION_2_8/2(AIB2)
  INTERSECTION_2_8/1(S1) -> [S_I_28]
  INTERSECTION_2_8/2(S2) -> [S_I_82]
  [BDB_2] -> INTERSECTION_2_8/3(BDB1)
  [BDB_8] -> INTERSECTION_2_8/4(BDB2)
  [control] -> INTERSECTION_2_8/5(control)
  [AIB_3] -> INTERSECTION_3_4/1(AIB1)
  [AIB_4] -> INTERSECTION_3_4/2(AIB2)
  INTERSECTION_3_4/1(S1) -> [S_I_34]
  INTERSECTION_3_4/2(S2) -> [S_I_43]
  [BDB_3] -> INTERSECTION_3_4/3(BDB1)
  [BDB_4] -> INTERSECTION_3_4/4(BDB2)
  [control] -> INTERSECTION_3_4/5(control)
  [AIB_3] -> INTERSECTION_3_5/1(AIB1)
  [AIB_5] -> INTERSECTION_3_5/2(AIB2)
  INTERSECTION_3_5/1(S1) -> [S_I_35]
  INTERSECTION_3_5/2(S2) -> [S_I_53]
  [BDB_3] -> INTERSECTION_3_5/3(BDB1)
  [BDB_5] -> INTERSECTION_3_5/4(BDB2)
  [control] -> INTERSECTION_3_5/5(control)
  [AIB_3] -> INTERSECTION_3_6/1(AIB1)
  [AIB_6] -> INTERSECTION_3_6/2(AIB2)
  INTERSECTION_3_6/1(S1) -> [S_I_36]
  INTERSECTION_3_6/2(S2) -> [S_I_63]
  [BDB_3] -> INTERSECTION_3_6/3(BDB1)
  [BDB_6] -> INTERSECTION_3_6/4(BDB2)
  [control] -> INTERSECTION_3_6/5(control)
  [AIB_3] -> INTERSECTION_3_7/1(AIB1)
  [AIB_7] -> INTERSECTION_3_7/2(AIB2)
  INTERSECTION_3_7/1(S1) -> [S_I_37]
  INTERSECTION_3_7/2(S2) -> [S_I_73]
  [BDB_3] -> INTERSECTION_3_7/3(BDB1)
  [BDB_7] -> INTERSECTION_3_7/4(BDB2)
  [control] -> INTERSECTION_3_7/5(control)
  [AIB_3] -> INTERSECTION_3_8/1(AIB1)
  [AIB_8] -> INTERSECTION_3_8/2(AIB2)
  INTERSECTION_3_8/1(S1) -> [S_I_38]
  INTERSECTION_3_8/2(S2) -> [S_I_83]
  [BDB_3] -> INTERSECTION_3_8/3(BDB1)
  [BDB_8] -> INTERSECTION_3_8/4(BDB2)
  [control] -> INTERSECTION_3_8/5(control)
  [AIB_3] -> INTERSECTION_3_9/1(AIB1)
  [AIB_9] -> INTERSECTION_3_9/2(AIB2)
  INTERSECTION_3_9/1(S1) -> [S_I_39]
  INTERSECTION_3_9/2(S2) -> [S_I_93]
  [BDB_3] -> INTERSECTION_3_9/3(BDB1)
  [BDB_9] -> INTERSECTION_3_9/4(BDB2)
  [control] -> INTERSECTION_3_9/5(control)
  [AIB_3] -> INTERSECTION_3_10/1(AIB1)
  [AIB_10] -> INTERSECTION_3_10/2(AIB2)
  INTERSECTION_3_10/1(S1) -> [S_I_310]
  INTERSECTION_3_10/2(S2) -> [S_I_103]
  [BDB_3] -> INTERSECTION_3_10/3(BDB1)
  [BDB_10] -> INTERSECTION_3_10/4(BDB2)
  [control] -> INTERSECTION_3_10/5(control)
  [AIB_4] -> INTERSECTION_4_5/1(AIB1)
  [AIB_5] -> INTERSECTION_4_5/2(AIB2)
  INTERSECTION_4_5/1(S1) -> [S_I_45]
  INTERSECTION_4_5/2(S2) -> [S_I_54]
  [BDB_4] -> INTERSECTION_4_5/3(BDB1)
  [BDB_5] -> INTERSECTION_4_5/4(BDB2)
  [control] -> INTERSECTION_4_5/5(control)
  [AIB_4] -> INTERSECTION_4_6/1(AIB1)
  [AIB_6] -> INTERSECTION_4_6/2(AIB2)
  INTERSECTION_4_6/1(S1) -> [S_I_46]
  INTERSECTION_4_6/2(S2) -> [S_I_64]
  [BDB_4] -> INTERSECTION_4_6/3(BDB1)
  [BDB_6] -> INTERSECTION_4_6/4(BDB2)
  [control] -> INTERSECTION_4_6/5(control)
  [AIB_4] -> INTERSECTION_4_7/1(AIB1)
  [AIB_7] -> INTERSECTION_4_7/2(AIB2)
  INTERSECTION_4_7/1(S1) -> [S_I_47]
  INTERSECTION_4_7/2(S2) -> [S_I_74]
  [BDB_4] -> INTERSECTION_4_7/3(BDB1)
  [BDB_7] -> INTERSECTION_4_7/4(BDB2)
  [control] -> INTERSECTION_4_7/5(control)
  [AIB_4] -> INTERSECTION_4_8/1(AIB1)
  [AIB_8] -> INTERSECTION_4_8/2(AIB2)
  INTERSECTION_4_8/1(S1) -> [S_I_48]
  INTERSECTION_4_8/2(S2) -> [S_I_84]
  [BDB_4] -> INTERSECTION_4_8/3(BDB1)
  [BDB_8] -> INTERSECTION_4_8/4(BDB2)
  [control] -> INTERSECTION_4_8/5(control)
  [AIB_4] -> INTERSECTION_4_9/1(AIB1)
  [AIB_9] -> INTERSECTION_4_9/2(AIB2)
  INTERSECTION_4_9/1(S1) -> [S_I_49]
  INTERSECTION_4_9/2(S2) -> [S_I_94]
  [BDB_4] -> INTERSECTION_4_9/3(BDB1)
  [BDB_9] -> INTERSECTION_4_9/4(BDB2)
  [control] -> INTERSECTION_4_9/5(control)
  [AIB_4] -> INTERSECTION_4_10/1(AIB1)
  [AIB_10] -> INTERSECTION_4_10/2(AIB2)
  INTERSECTION_4_10/1(S1) -> [S_I_410]
  INTERSECTION_4_10/2(S2) -> [S_I_104]
  [BDB_4] -> INTERSECTION_4_10/3(BDB1)
  [BDB_10] -> INTERSECTION_4_10/4(BDB2)
  [control] -> INTERSECTION_4_10/5(control)
  [AIB_5] -> INTERSECTION_5_6/1(AIB1)
  [AIB_6] -> INTERSECTION_5_6/2(AIB2)
  INTERSECTION_5_6/1(S1) -> [S_I_56]
  INTERSECTION_5_6/2(S2) -> [S_I_65]
  [BDB_5] -> INTERSECTION_5_6/3(BDB1)
  [BDB_6] -> INTERSECTION_5_6/4(BDB2)
  [control] -> INTERSECTION_5_6/5(control)
  [AIB_5] -> INTERSECTION_5_7/1(AIB1)
  [AIB_7] -> INTERSECTION_5_7/2(AIB2)
  INTERSECTION_5_7/1(S1) -> [S_I_57]
  INTERSECTION_5_7/2(S2) -> [S_I_75]
  [BDB_5] -> INTERSECTION_5_7/3(BDB1)
  [BDB_7] -> INTERSECTION_5_7/4(BDB2)
  [control] -> INTERSECTION_5_7/5(control)
  [AIB_5] -> INTERSECTION_5_8/1(AIB1)
  [AIB_8] -> INTERSECTION_5_8/2(AIB2)
  INTERSECTION_5_8/1(S1) -> [S_I_58]
  INTERSECTION_5_8/2(S2) -> [S_I_85]
  [BDB_5] -> INTERSECTION_5_8/3(BDB1)
  [BDB_8] -> INTERSECTION_5_8/4(BDB2)
  [control] -> INTERSECTION_5_8/5(control)
  [AIB_5] -> INTERSECTION_5_9/1(AIB1)
  [AIB_9] -> INTERSECTION_5_9/2(AIB2)
  INTERSECTION_5_9/1(S1) -> [S_I_59]
  INTERSECTION_5_9/2(S2) -> [S_I_95]
  [BDB_5] -> INTERSECTION_5_9/3(BDB1)
  [BDB_9] -> INTERSECTION_5_9/4(BDB2)
  [control] -> INTERSECTION_5_9/5(control)
  [AIB_5] -> INTERSECTION_5_10/1(AIB1)
  [AIB_10] -> INTERSECTION_5_10/2(AIB2)
  INTERSECTION_5_10/1(S1) -> [S_I_510]
  INTERSECTION_5_10/2(S2) -> [S_I_105]
  [BDB_5] -> INTERSECTION_5_10/3(BDB1)
  [BDB_10] -> INTERSECTION_5_10/4(BDB2)
  [control] -> INTERSECTION_5_10/5(control)
  [AIB_6] -> INTERSECTION_6_7/1(AIB1)
  [AIB_7] -> INTERSECTION_6_7/2(AIB2)
  INTERSECTION_6_7/1(S1) -> [S_I_67]
  INTERSECTION_6_7/2(S2) -> [S_I_76]
  [BDB_6] -> INTERSECTION_6_7/3(BDB1)
  [BDB_7] -> INTERSECTION_6_7/4(BDB2)
  [control] -> INTERSECTION_6_7/5(control)
  [AIB_6] -> INTERSECTION_6_8/1(AIB1)
  [AIB_8] -> INTERSECTION_6_8/2(AIB2)
  INTERSECTION_6_8/1(S1) -> [S_I_68]
  INTERSECTION_6_8/2(S2) -> [S_I_86]
  [BDB_6] -> INTERSECTION_6_8/3(BDB1)
  [BDB_8] -> INTERSECTION_6_8/4(BDB2)
  [control] -> INTERSECTION_6_8/5(control)
  [AIB_6] -> INTERSECTION_6_9/1(AIB1)
  [AIB_9] -> INTERSECTION_6_9/2(AIB2)
  INTERSECTION_6_9/1(S1) -> [S_I_69]
  INTERSECTION_6_9/2(S2) -> [S_I_96]
  [BDB_6] -> INTERSECTION_6_9/3(BDB1)
  [BDB_9] -> INTERSECTION_6_9/4(BDB2)
  [control] -> INTERSECTION_6_9/5(control)
  [AIB_6] -> INTERSECTION_6_10/1(AIB1)
  [AIB_10] -> INTERSECTION_6_10/2(AIB2)
  INTERSECTION_6_10/1(S1) -> [S_I_610]
  INTERSECTION_6_10/2(S2) -> [S_I_106]
  [BDB_6] -> INTERSECTION_6_10/3(BDB1)
  [BDB_10] -> INTERSECTION_6_10/4(BDB2)
  [control] -> INTERSECTION_6_10/5(control)
  [AIB_7] -> INTERSECTION_7_8/1(AIB1)
  [AIB_8] -> INTERSECTION_7_8/2(AIB2)
  INTERSECTION_7_8/1(S1) -> [S_I_78]
  INTERSECTION_7_8/2(S2) -> [S_I_87]
  [BDB_7] -> INTERSECTION_7_8/3(BDB1)
  [BDB_8] -> INTERSECTION_7_8/4(BDB2)
  [control] -> INTERSECTION_7_8/5(control)
  [AIB_7] -> INTERSECTION_7_9/1(AIB1)
  [AIB_9] -> INTERSECTION_7_9/2(AIB2)
  INTERSECTION_7_9/1(S1) -> [S_I_79]
  INTERSECTION_7_9/2(S2) -> [S_I_97]
  [BDB_7] -> INTERSECTION_7_9/3(BDB1)
  [BDB_9] -> INTERSECTION_7_9/4(BDB2)
  [control] -> INTERSECTION_7_9/5(control)
  [AIB_7] -> INTERSECTION_7_10/1(AIB1)
  [AIB_10] -> INTERSECTION_7_10/2(AIB2)
  INTERSECTION_7_10/1(S1) -> [S_I_710]
  INTERSECTION_7_10/2(S2) -> [S_I_107]
  [BDB_7] -> INTERSECTION_7_10/3(BDB1)
  [BDB_10] -> INTERSECTION_7_10/4(BDB2)
  [control] -> INTERSECTION_7_10/5(control)
  [AIB_8] -> INTERSECTION_8_9/1(AIB1)
  [AIB_9] -> INTERSECTION_8_9/2(AIB2)
  INTERSECTION_8_9/1(S1) -> [S_I_89]
  INTERSECTION_8_9/2(S2) -> [S_I_98]
  [BDB_8] -> INTERSECTION_8_9/3(BDB1)
  [BDB_9] -> INTERSECTION_8_9/4(BDB2)
  [control] -> INTERSECTION_8_9/5(control)
  [AIB_8] -> INTERSECTION_8_10/1(AIB1)
  [AIB_10] -> INTERSECTION_8_10/2(AIB2)
  INTERSECTION_8_10/1(S1) -> [S_I_810]
  INTERSECTION_8_10/2(S2) -> [S_I_108]
  [BDB_8] -> INTERSECTION_8_10/3(BDB1)
  [BDB_10] -> INTERSECTION_8_10/4(BDB2)
  [control] -> INTERSECTION_8_10/5(control)
  [AIB_9] -> INTERSECTION_9_10/1(AIB1)
  [AIB_10] -> INTERSECTION_9_10/2(AIB2)
  INTERSECTION_9_10/1(S1) -> [S_I_910]
  INTERSECTION_9_10/2(S2) -> [S_I_109]
  [BDB_9] -> INTERSECTION_9_10/3(BDB1)
  [BDB_10] -> INTERSECTION_9_10/4(BDB2)
  [control] -> INTERSECTION_9_10/5(control)
  ZONE_1/1(BDB) -> [BDB_1]
  ZONE_1/2(AIB) -> [AIB_1]
  ZONE_1/3(theta_out) -> [theta_out_1z]
  [qdot_in_1] -> ZONE_1/5(Qdot_in)
  [S_in_1] -> ZONE_1/4(S_in)
  [GDB] -> ZONE_1/2(GDB)
  [NDB] -> ZONE_1/3(NDB)
  [control] -> ZONE_1/6(control)
  [WDB] -> ZONE_1/1(WDB)

== system building_EXAMPLE_v1/DATALOGGER ==
  WDB : Inport
  GDB : Inport  Port=2
  NDB : Inport  Port=3
  AIB_z1 : Inport  Port=4
  AIB_z2 : Inport  Port=5
  AIB_z3 : Inport  Port=6
  AIB_z4 : Inport  Port=7
  AIB_z5 : Inport  Port=8
  AIB_z6 : Inport  Port=9
  AIB_z7 : Inport  Port=10
  AIB_z8 : Inport  Port=11
  AIB_z9 : Inport  Port=12
  AIB_z10 : Inport  Port=13
  BDB_z1 : Inport  Port=14
  BDB_z2 : Inport  Port=15
  BDB_z3 : Inport  Port=16
  BDB_z4 : Inport  Port=17
  BDB_z5 : Inport  Port=18
  BDB_z6 : Inport  Port=19
  BDB_z7 : Inport  Port=20
  BDB_z8 : Inport  Port=21
  BDB_z9 : Inport  Port=22
  BDB_z10 : Inport  Port=23
  HVAC : Inport  Port=24
  datalogger : Inport  Port=25
  AIBz1 : Subsystem
  AIBz10 : Subsystem
  AIBz2 : Subsystem
  AIBz3 : Subsystem
  AIBz4 : Subsystem
  AIBz5 : Subsystem
  AIBz6 : Subsystem
  AIBz7 : Subsystem
  AIBz8 : Subsystem
  AIBz9 : Subsystem
  Bus Creator : BusCreator  Inputs=10
  Bus Creator1 : BusCreator  Inputs=10
  Bus Creator2 : BusCreator  Inputs=3
  logger_AIB : Subsystem
  logger_BDB : Subsystem
  logger_BOUNDARY : Subsystem
  logger_HVAC : Subsystem
  z1 : Subsystem
  z10 : Subsystem
  z2 : Subsystem
  z3 : Subsystem
  z4 : Subsystem
  z5 : Subsystem
  z6 : Subsystem
  z7 : Subsystem
  z8 : Subsystem
  z9 : Subsystem
  wires:
  WDB/1 -> Bus Creator2/1
  Bus Creator/1 -> logger_AIB/1(AIB)
  datalogger/1 -> logger_BOUNDARY/Enable, logger_AIB/Enable, logger_BDB/Enable, logger_HVAC/Enable
  GDB/1 -> Bus Creator2/2
  NDB/1 -> Bus Creator2/3
  AIB_z1/1 -> AIBz1/1(AIB)
  Bus Creator1/1 -> logger_BDB/1(BDB)
  Bus Creator2/1 -> logger_BOUNDARY/1(BOUNDARY)
  BDB_z1/1 -> z1/1(BDB)
  z1/1(BDB') -> Bus Creator1/1  "z1"
  BDB_z2/1 -> z2/1(BDB)
  z2/1(BDB') -> Bus Creator1/2  "z2"
  z3/1(BDB') -> Bus Creator1/3  "z3"
  BDB_z3/1 -> z3/1(BDB)
  BDB_z4/1 -> z4/1(BDB)
  z4/1(BDB') -> Bus Creator1/4  "z4"
  BDB_z5/1 -> z5/1(BDB)
  z5/1(BDB') -> Bus Creator1/5  "z5"
  BDB_z6/1 -> z6/1(BDB)
  z6/1(BDB') -> Bus Creator1/6  "z6"
  BDB_z7/1 -> z7/1(BDB)
  z7/1(BDB') -> Bus Creator1/7  "z7"
  BDB_z8/1 -> z8/1(BDB)
  z8/1(BDB') -> Bus Creator1/8  "z8"
  BDB_z9/1 -> z9/1(BDB)
  z9/1(BDB') -> Bus Creator1/9  "z9"
  BDB_z10/1 -> z10/1(BDB)
  z10/1(BDB') -> Bus Creator1/10  "z10"
  AIBz1/1(AIB') -> Bus Creator/1  "z1"
  AIBz2/1(AIB') -> Bus Creator/2  "z2"
  AIB_z2/1 -> AIBz2/1(AIB)
  AIB_z3/1 -> AIBz3/1(AIB)
  AIBz3/1(AIB') -> Bus Creator/3  "z3"
  AIB_z4/1 -> AIBz4/1(AIB)
  AIBz4/1(AIB') -> Bus Creator/4  "z4"
  AIB_z5/1 -> AIBz5/1(AIB)
  AIBz5/1(AIB') -> Bus Creator/5  "z5"
  AIB_z6/1 -> AIBz6/1(AIB)
  AIBz6/1(AIB') -> Bus Creator/6  "z6"
  AIB_z7/1 -> AIBz7/1(AIB)
  AIBz7/1(AIB') -> Bus Creator/7  "z7"
  AIB_z8/1 -> AIBz8/1(AIB)
  AIBz8/1(AIB') -> Bus Creator/8  "z8"
  AIB_z9/1 -> AIBz9/1(AIB)
  AIBz9/1(AIB') -> Bus Creator/9  "z9"
  AIB_z10/1 -> AIBz10/1(AIB)
  AIBz10/1(AIB') -> Bus Creator/10  "z10"
  HVAC/1 -> logger_HVAC/1(HVAC)
